simulink model "flatearthsixdof"  (R2025a)
settings: Solver=FixedStepAuto  StartTime=0.0  StopTime=90  FixedStep=0.01  RelTol=1e-3
model workspace (MAT data in the model file):
  aero_data.Mach = [0.01 0.02 0.03 0.04 0.05 0.06 0.07 0.08 0.09 0.1 0.11 0.12 ... (7499 elements, 7499x1)]
  aero_data.Alpha = [0 0 0 0 0 0 0 0 0 0 0 0 ... (7499 elements, 7499x1)]
  aero_data.CD = [0.376420475734 0.37891218399 0.374582423788 0.370163231763 0.366269784455 0.362896739037 0.359959262302 0.357376271103 0.355082207872 0.35302595791 0.351167736032 0.349476360929 ... (7499 elements, 7499x1)]
  aero_data.CL = [0 0 0 0 0 0 0 0 0 0 0 0 ... (7499 elements, 7499x1)]
  aero_data.CP = [3.54714585938 3.54714585938 3.54714585938 3.54714585938 3.54714585938 3.54714585938 3.54714585938 3.54714585938 3.54714585938 3.54714585938 3.54714585938 3.54714585938 ... (7499 elements, 7499x1)]
  aero_data.CNalpha = [4.21136352134 4.21136352134 4.21136352134 4.21136352134 4.21136352134 4.21136352134 4.21136352134 4.21136352134 4.21136352134 4.21136352134 4.21136352134 4.21136352134 ... (7499 elements, 7499x1)]
  aero_data.Cm_alpha = [7.59260560273 7.59260560273 7.59260560273 7.59260560273 7.59260560273 7.59260560273 7.59260560273 7.59260560273 7.59260560273 7.59260560273 7.59260560273 7.59260560273 ... (7499 elements, 7499x1)]
  d_body_mc = 0.4
  designFocus = "reference-tracking"
  drydenSeed_mc = [23341 23342 23343 23344]
  m_initial_mc = [0 20 25 25 20 25 70 1 10 15 1 20 120 1 50 5 1 5 5 10 10]
  schedule(1).Mach_grid = 0
  schedule(1).Kp = 0.0539603522173
  schedule(1).Kd = 0.0467310358173
  schedule(1).Ts = 0.0389337885936
  schedule(2).Mach_grid = 0.1
  schedule(2).Kp = 0.0926620388775
  schedule(2).Kd = 0.0630517482841
  schedule(2).Ts = 0.0389337885936
  schedule(3).Mach_grid = 0.2
  schedule(3).Kp = 0.148668674318
  schedule(3).Kd = 0.0833093726921
  schedule(3).Ts = 0.0389337885936
  schedule(4).Mach_grid = 0.3
  schedule(4).Kp = 0.224059304208
  schedule(4).Kd = 0.106722577169
  schedule(4).Ts = 0.0389337885936
  schedule(5).Mach_grid = 0.4
  schedule(5).Kp = 1.96086663664
  schedule(5).Kd = 0.812163631669
  schedule(5).Ts = 0.0389337885936
  schedule(6).Mach_grid = 0.5
  schedule(6).Kp = 2.40062252085
  schedule(6).Kd = 0.879576960286
  schedule(6).Ts = 0.0389337885936
  schedule(7).Mach_grid = 0.6
  schedule(7).Kp = 2.80522895598
  schedule(7).Kd = 0.92149637698
  schedule(7).Ts = 0.0389337885936
  schedule(8).Mach_grid = 0.7
  schedule(8).Kp = 3.14273502179
  schedule(8).Kd = 0.935580375892
  schedule(8).Ts = 0.0389337885936
  schedule(9).Mach_grid = 0.8
  schedule(9).Kp = 1.01599465816
  schedule(9).Kd = 0.276532829281
  schedule(9).Ts = 0.0389337885936
  schedule(10).Mach_grid = 0.9
  schedule(10).Kp = 3.37328201224
  schedule(10).Kd = 0.845653344317
  schedule(10).Ts = 0.0389337885936
  schedule(11).Mach_grid = 1
  schedule(11).Kp = 2.87563806108
  schedule(11).Kd = 0.668149554703
  schedule(11).Ts = 0.0389337885936
  schedule(12).Mach_grid = 1.1
  schedule(12).Kp = 2.15595228552
  schedule(12).Kd = 0.466777362151
  schedule(12).Ts = 0.0389337885936
  x_mc = [0 0.3 0.7 1.1 1.2 2.2 2.3 2.9 3.1 3.3 3.4 4 4.2 4.3 4.9 6 6.5 6.7 6.9 7.1 7.6]
undefined symbols (not defined in the file or in its folder): F, Light, MIL
libraries: simulink_extras x6, aerolibutil x2, aerolibwind2 x1, aerolibatmos2 x1
settings Model: Creator=rog  LastModifiedBy=rog

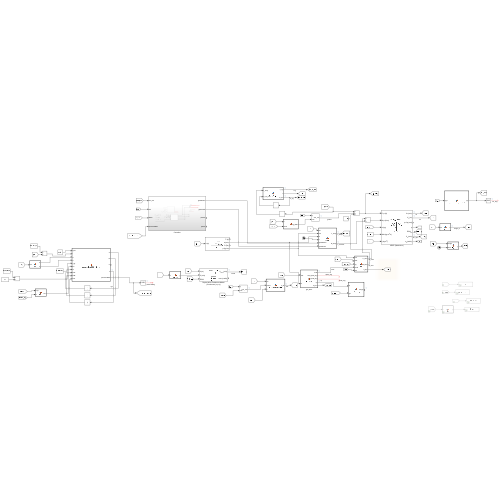
[thumbnail: Simulink's stored preview of the top-level diagram]
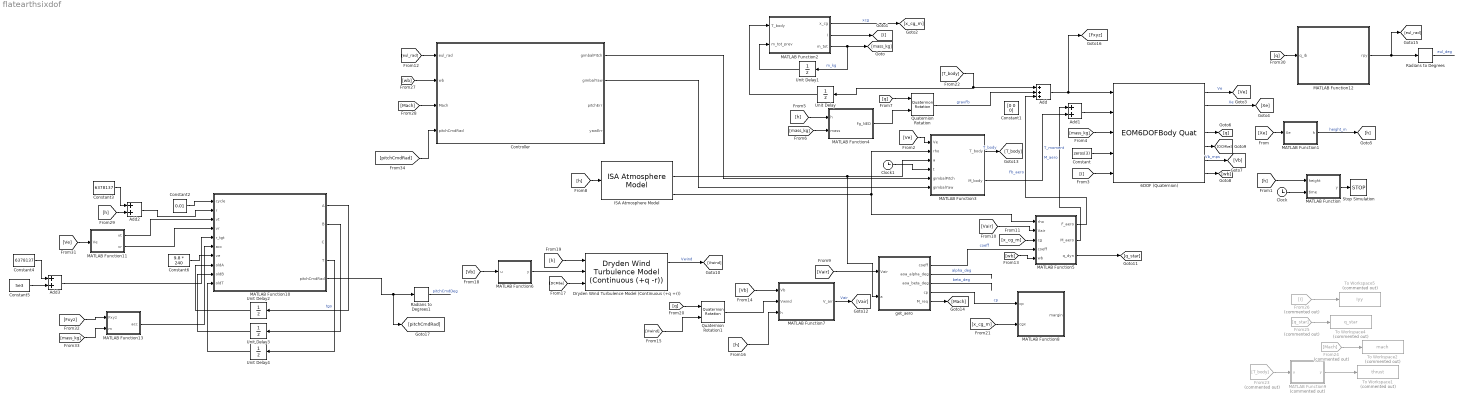
== system flatearthsixdof ==
  6DOF (Quaternion) : EOM6DOFBodyQuat  mtype=Custom Variable  Vm_0=[0.1 0 0]  eul_0=[0 deg2rad(90) 0]
  Add : Sum  Inputs=+++
  Add1 : Sum
  Add2 : Sum
  Add3 : Sum
  Clock : Clock
  Clock1 : Clock
  Constant : Constant  Value=zeros(3)
  Constant1 : Constant  Value=[0 0 0]
  Constant2 : Constant  Value=0.01
  Constant3 : Constant  Value=6378137
  Constant4 : Constant  Value=6378137
  Constant5 : Constant  Value=5e3
  Constant6 : Constant  Value=9.8 * 240
  Controller : Subsystem
  Dryden Wind Turbulence Model (Continuous (+q +r)) : aerolibwind2/Dryden Wind Turbulence Model  (Continuous (+q -r))  units=Metric (MKS)  spec=MIL-F-8785C  model=Continuous Dryden (+q +r)  W20=15  Wdeg=0  TurbProb=10^-2 - Light  L_high=533.4  Wingspan=10  ts=0.1  Seed=drydenSeed_mc  T_on=on
      settings: LibrarySourceBlock=|
      | aerolibwind2/Dryden Wind Turbulence Model
      | (Continuous (+q +r))
  From23 : From  Commented=on  GotoTag=T_body
  From24 : From  Commented=on  GotoTag=Mach
  From25 : From  Commented=on  GotoTag=q_star
  From26 : From  Commented=on  GotoTag=I
  ISA Atmosphere Model : aerolibatmos2/ISA Atmosphere Model  useExtended=on  action=Warning  custom=off  viscosityOut=off  g=9.80665  gamma=1.4  R=287.0531  L=0.0065  h_trop=11000  h_strat=20000  rho0=1.225  P0=101325  T0=288.15  h0=0  S=110.4  Tref=273.15  muref=1.716e-5
  MATLAB Function : MATLAB Function  TreatAsAtomicUnit=on
  MATLAB Function1 : MATLAB Function  TreatAsAtomicUnit=on
  MATLAB Function10 : MATLAB Function  TreatAsAtomicUnit=on
  MATLAB Function11 : MATLAB Function  TreatAsAtomicUnit=on
  MATLAB Function12 : MATLAB Function  TreatAsAtomicUnit=on
  MATLAB Function13 : MATLAB Function  TreatAsAtomicUnit=on
  MATLAB Function2 : MATLAB Function  TreatAsAtomicUnit=on
  MATLAB Function3 : MATLAB Function  TreatAsAtomicUnit=on
  MATLAB Function4 : MATLAB Function  TreatAsAtomicUnit=on
  MATLAB Function5 : MATLAB Function  TreatAsAtomicUnit=on
  MATLAB Function6 : MATLAB Function  TreatAsAtomicUnit=on
  MATLAB Function7 : MATLAB Function  TreatAsAtomicUnit=on
  MATLAB Function8 : MATLAB Function  TreatAsAtomicUnit=on
  MATLAB Function9 : MATLAB Function  Commented=on  TreatAsAtomicUnit=on
  Quaternion Rotation : aerolibutil/Quaternion Rotation
  Quaternion Rotation1 : aerolibutil/Quaternion Rotation
  Radians to Degrees : simulink_extras/Transformations/Radians to Degrees
  Radians to Degrees1 : simulink_extras/Transformations/Radians to Degrees
  Stop Simulation : Stop
  To Workspace1 : ToWorkspace  Commented=on  VariableName=thrust  SaveFormat=Timeseries  SampleTime=-1
  To Workspace2 : ToWorkspace  Commented=on  VariableName=mach  SaveFormat=Timeseries  SampleTime=-1
  To Workspace4 : ToWorkspace  Commented=on  VariableName=q_star  SaveFormat=Timeseries  SampleTime=-1
  To Workspace5 : ToWorkspace  Commented=on  VariableName=Iyy  SaveFormat=Timeseries  SampleTime=-1
  Unit Delay : UnitDelay  InitialCondition=[0 0 0]  SampleTime=-1  HasFrameUpgradeWarning=on
  Unit Delay1 : UnitDelay  InitialCondition=439  SampleTime=-1  HasFrameUpgradeWarning=on
  Unit Delay2 : UnitDelay  SampleTime=-1  HasFrameUpgradeWarning=on
  Unit Delay3 : UnitDelay  SampleTime=-1  HasFrameUpgradeWarning=on
  Unit Delay4 : UnitDelay  InitialCondition=90  SampleTime=-1  HasFrameUpgradeWarning=on
  get_aero : MATLAB Function  TreatAsAtomicUnit=on
  wires:
  Constant/1 -> 6DOF (Quaternion)/4
  MATLAB Function/1(y) -> Stop Simulation/1
  Clock/1 -> MATLAB Function/2(time)
  MATLAB Function2/2(I) -> [I]
  MATLAB Function2/1(x_cg) -> [x_cg_m]  "xcg"
  MATLAB Function2/3(m_tot) -> Unit Delay1/1, [mass_kg]  "m_kg"
  6DOF (Quaternion)/1 -> [Ve]  "Ve"
  6DOF (Quaternion)/2 -> [Xe]  "Xe"
  [h] -> MATLAB Function/1(height)
  [Xe] -> MATLAB Function1/1(Xe)
  MATLAB Function1/1(h) -> [h]  "height_m"
  [Ve] -> MATLAB Function3/1(Ve)
  [I] -> 6DOF (Quaternion)/5
  [mass_kg] -> 6DOF (Quaternion)/3
  Add/1 -> [Fxyz], 6DOF (Quaternion)/1
  [h] -> MATLAB Function4/1(h)
  [mass_kg] -> MATLAB Function4/2(mass)
  6DOF (Quaternion)/4 -> [q]
  [q] -> Quaternion Rotation/1
  MATLAB Function4/1(Fg_NED) -> Quaternion Rotation/2
  Quaternion Rotation/1 -> Add/2  "gravFb"
  [h] -> ISA Atmosphere Model/1
  Clock1/1 -> MATLAB Function3/4(t)
  6DOF (Quaternion)/6 -> [Vb]  "Vb_mps"
  ISA Atmosphere Model/2 -> get_aero/2(a), MATLAB Function3/3(a)
  get_aero/1(coeff) -> MATLAB Function5/4(coeff)  "coeff"
  [x_cg_m] -> MATLAB Function5/3(cg)
  Radians to Degrees/1 -> ?  "eul_deg"
  get_aero/2(aoa_alpha_deg) -> ?  "alpha_deg"
  get_aero/3(aoa_beta_deg) -> ?  "beta_deg"
  [wb] -> MATLAB Function5/5(wb)
  6DOF (Quaternion)/7 -> [wb]
  Unit Delay/1 -> MATLAB Function2/1(T_body)
  ISA Atmosphere Model/4 -> MATLAB Function5/1(rho), MATLAB Function3/2(rho)
  6DOF (Quaternion)/5 -> [DCMbe]
  [h] -> Dryden Wind Turbulence Model (Continuous (+q +r))/1
  MATLAB Function6/1(y) -> Dryden Wind Turbulence Model (Continuous (+q +r))/2
  [DCMbe] -> Dryden Wind Turbulence Model (Continuous (+q +r))/3
  [Vb] -> MATLAB Function6/1(u)
  Dryden Wind Turbulence Model (Continuous (+q +r))/1 -> [Vwind]  "Vwind"
  [Vb] -> MATLAB Function7/1(Vb)
  Quaternion Rotation1/1 -> MATLAB Function7/2(Vwind)
  MATLAB Function7/1(V_air) -> [Vair]  "Vair"
  [Vwind] -> Quaternion Rotation1/2
  [q] -> Quaternion Rotation1/1
  Unit Delay1/1 -> MATLAB Function2/2(m_tot_prev)
  get_aero/4(cp) -> MATLAB Function8/1(cp)  "cp"
  MATLAB Function5/1(F_aero) -> Add/3  "Fb_aero"
  [Vair] -> get_aero/1(Vair)
  [Vair] -> MATLAB Function5/2(Vair)
  [h] -> MATLAB Function7/3(h)
  [x_cg_m] -> MATLAB Function8/2(cgx)
  MATLAB Function5/3(q_dyn) -> [q_star]
  From25/1 -> To Workspace4/1
  From26/1 -> To Workspace5/1
  MATLAB Function3/1(T_body) -> [T_body]  "T_body"
  [T_body] -> Unit Delay/1, Add/1
  From23/1 -> MATLAB Function9/1(u)
  MATLAB Function9/1(y) -> To Workspace1/1
  get_aero/5(M_req) -> [Mach]
  From24/1 -> To Workspace2/1
  Add1/1 -> 6DOF (Quaternion)/2
  MATLAB Function3/2(M_body) -> Add1/2  "T_moment"
  [q] -> MATLAB Function12/1(q_ib)
  MATLAB Function12/1(rpy) -> [eul_rad], Radians to Degrees/1
  MATLAB Function5/2(M_aero) -> Add1/1  "M_aero"
  Controller/1(gimbalPitch) -> MATLAB Function3/5(gimbalPitch)
  Controller/2(gimbalYaw) -> MATLAB Function3/6(gimbalYaw)
  [eul_rad] -> Controller/1(eul_rad)
  [wb] -> Controller/2(wb)
  [Mach] -> Controller/3(Mach)
  MATLAB Function10/1(A) -> Unit Delay2/1
  MATLAB Function10/2(B) -> Unit Delay3/1
  MATLAB Function10/4(T) -> Unit Delay4/1  "tgo"
  Unit Delay4/1 -> MATLAB Function10/10(oldT)
  Unit Delay3/1 -> MATLAB Function10/9(oldB)
  Unit Delay2/1 -> MATLAB Function10/8(oldA)
  Constant2/1 -> MATLAB Function10/1(cycle)
  Constant3/1 -> Add2/1
  [h] -> Add2/2
  Add2/1 -> MATLAB Function10/2(r)
  [Ve] -> MATLAB Function11/1(Ve)
  MATLAB Function11/1(vt) -> MATLAB Function10/3(vt)
  MATLAB Function11/2(vr) -> MATLAB Function10/4(vr)
  Constant5/1 -> Add3/2
  Constant4/1 -> Add3/1
  Add3/1 -> MATLAB Function10/5(r_tgt)
  Constant6/1 -> MATLAB Function10/7(ve)
  [Fxyz] -> MATLAB Function13/1(Fxyz)
  [mass_kg] -> MATLAB Function13/2(m)
  MATLAB Function13/1(acc) -> MATLAB Function10/6(acc)
  MATLAB Function10/5(pitchCmdRad) -> [pitchCmdRad], Radians to Degrees1/1
  Radians to Degrees1/1 -> ?  "pitchCmdDeg"
  [pitchCmdRad] -> Controller/4(pitchCmdRad)

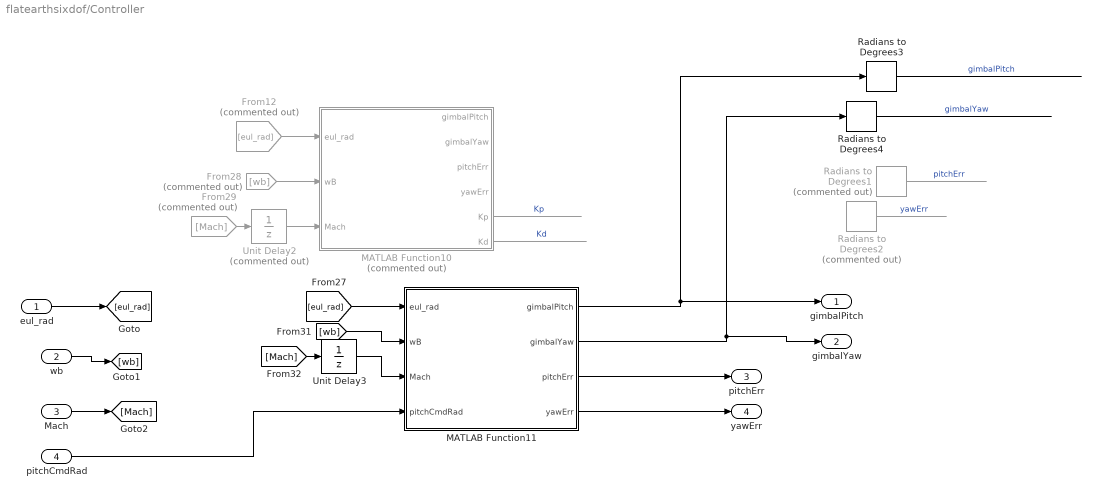
== system flatearthsixdof/Controller ==
  eul_rad : Inport
  wb : Inport  Port=2
  Mach : Inport  Port=3
  pitchCmdRad : Inport  Port=4
  From12 : From  Commented=on  GotoTag=eul_rad
  From28 : From  Commented=on  GotoTag=wb
  From29 : From  Commented=on  GotoTag=Mach
  MATLAB Function10 : MATLAB Function  Commented=on  TreatAsAtomicUnit=on
  MATLAB Function11 : MATLAB Function  TreatAsAtomicUnit=on
  Radians to Degrees1 : simulink_extras/Transformations/Radians to Degrees  Commented=on
  Radians to Degrees2 : simulink_extras/Transformations/Radians to Degrees  Commented=on
  Radians to Degrees3 : simulink_extras/Transformations/Radians to Degrees
  Radians to Degrees4 : simulink_extras/Transformations/Radians to Degrees
  Unit Delay2 : UnitDelay  Commented=on  SampleTime=-1  HasFrameUpgradeWarning=on
  Unit Delay3 : UnitDelay  SampleTime=-1  HasFrameUpgradeWarning=on
  gimbalPitch : Outport
  gimbalYaw : Outport  Port=2
  pitchErr : Outport  Port=3
  yawErr : Outport  Port=4
  wires:
  From28/1 -> MATLAB Function10/2(wB)
  Radians to Degrees1/1 -> ?  "pitchErr"
  From12/1 -> MATLAB Function10/1(eul_rad)
  Radians to Degrees3/1 -> ?  "gimbalPitch"
  [Mach] -> Unit Delay3/1
  Radians to Degrees2/1 -> ?  "yawErr"
  From29/1 -> Unit Delay2/1
  MATLAB Function10/6(Kd) -> ?  "Kd"
  Unit Delay2/1 -> MATLAB Function10/3(Mach)
  [wb] -> MATLAB Function11/2(wB)
  [eul_rad] -> MATLAB Function11/1(eul_rad)
  MATLAB Function11/2(gimbalYaw) -> Radians to Degrees4/1, gimbalYaw/1
  Unit Delay3/1 -> MATLAB Function11/3(Mach)
  Radians to Degrees4/1 -> ?  "gimbalYaw"
  MATLAB Function11/4(yawErr) -> yawErr/1
  MATLAB Function10/5(Kp) -> ?  "Kp"
  MATLAB Function11/3(pitchErr) -> pitchErr/1
  Mach/1 -> [Mach]
  wb/1 -> [wb]
  eul_rad/1 -> [eul_rad]
  pitchCmdRad/1 -> MATLAB Function11/4(pitchCmdRad)
  MATLAB Function11/1(gimbalPitch) -> gimbalPitch/1, Radians to Degrees3/1

== matlab function flatearthsixdof/MATLAB Function6 ==
  data: u input; y output
function y = twonorm(u)

y = norm(u);

== matlab function flatearthsixdof/get_aero ==
  data: Vair input size=[3 1]; coeff output; a input; aoa_alpha_deg output; aoa_beta_deg output; cp output; M_req output
function [coeff, aoa_alpha_deg, aoa_beta_deg, cp, M_req] = get_aero(Vair, a)

    u = Vair(1);
    v = Vair(2);
    w = Vair(3);

    V = sqrt(u*u + v*v + w*w);

    if V < 1e-6
        coeff = zeros(4,1);
        aoa_alpha_deg = 0;
        aoa_beta_deg  = 0;
        cp = 0;
        M_req = 0;
        return;
    end

    % Alpha / beta
    alpha = atan2(w, u);
    Vxz   = sqrt(u*u + w*w);

    if Vxz < 1e-6
        beta = 0;
    else
        beta = atan2(v, Vxz);
    end

    alpha_deg = alpha * 180/pi;
    beta_deg  = beta  * 180/pi;

    aoa_alpha_deg = alpha_deg;
    aoa_beta_deg  = beta_deg;

    % Total angle for drag & CP
    alpha_t = atan2( sqrt(v*v + w*w), u );
    aoa_t_deg = alpha_t * 180/pi;

    M_req = V / a;

    % Load aero once
    persistent aero
    if isempty(aero)
        S = load("aero.mat");
        aero = S.aero_data;
    end

    Alpha   = aero.Alpha;
    Mach    = aero.Mach;
    CD_full = aero.CD;
    CL_full = aero.CL;
    CP_full = aero.CP;

    % Lift from alpha & beta (same symmetric table)
    [~, CLa, ~] = lookup_coeff_nearest(alpha_deg, M_req, Alpha, Mach, CD_full, CL_full, CP_full);
    [~, CLb, ~] = lookup_coeff_nearest(beta_deg,  M_req, Alpha, Mach, CD_full, CL_full, CP_full);

    % Drag + CP from total angle
    [CD, ~, CP] = lookup_coeff_nearest(aoa_t_deg, M_req, Alpha, Mach, CD_full, CL_full, CP_full);

    cp = CP;

    coeff = [CD; CLa; CLb; CP];
end


function [cd, cl, cp] = lookup_coeff(aoa_deg, M_req, ...
                                     Alpha, Mach, CD_full, CL_full, CP_full)

    [~, iMach] = min(abs(Mach - M_req));
    Mach_near  = Mach(iMach);

    rows = find(abs(Mach - Mach_near) < 1e-6);

    A_slice  = Alpha(rows);
    CD_slice = CD_full(rows);
    CL_slice = CL_full(rows);
    CP_slice = CP_full(rows);

    cd = interp1(A_slice, CD_slice, aoa_deg, "linear", "extrap");
    cl = interp1(A_slice, CL_slice, aoa_deg, "linear", "extrap");
    cp = interp1(A_slice, CP_slice, aoa_deg, "linear", "extrap");
end


function [cd, cl, cp] = lookup_coeff_nearest(aoa_deg, M_req, ...
                                             Alpha, Mach, CD_full, CL_full, CP_full)

    [~, iMach] = min(abs(Mach - M_req));
    Mach_near  = Mach(iMach);

    rows = find(abs(Mach - Mach_near) < 1e-6);

    A_slice = Alpha(rows);

    [~, k] = min(abs(A_slice - aoa_deg));
    idx    = rows(k);

    cd = CD_full(idx);
    cl = CL_full(idx);
    cp = CP_full(idx);
end

== matlab function flatearthsixdof/MATLAB Function8 ==
  data: cp input; margin output; cgx input; d_body_mc parameter
function margin  = stabilitymargin(cp, cgx, d_body_mc)


margin = (cp-cgx)/d_body_mc;

== matlab function flatearthsixdof/MATLAB Function9 ==
  data: u input; y output
function y = fcn(u)

y = norm(u);

== matlab function flatearthsixdof/Controller/MATLAB Function10 ==
  data: eul_rad input; gimbalPitch output; wB input; Mach input; gimbalYaw output; pitchErr output; yawErr output; schedule parameter; Kp output; Kd output
function [gimbalPitch, gimbalYaw, pitchErr, yawErr, Kp, Kd] = tvc_gainsched_eulXYZ_pd(eul_rad, wB, Mach, schedule)
% Gain-scheduled TVC PD controller using Euler attitude error (XYZ order).
% eul_rad is assumed to be Euler angles RELATIVE TO THE VERTICAL reference,
% so the desired attitude corresponds to eul_rad = [0;0;0] (or [0 0 0]).
%
% Euler order: XYZ
%   eul_rad(1) = roll  about body +X
%   eul_rad(2) = pitch about body +Y
%   eul_rad(3) = yaw   about body +Z
%
% Control uses pitch and yaw only:
%   pitchErr = eul_rad(2), yawErr = eul_rad(3)
% D term uses measured body rates:
%   q_rate = wB(2), r_rate = wB(3)

%% ----- USER LIMITS -----
gimbalLimit = deg2rad(6);

%% ----- Gain schedule (nearest Mach) -----
n = numel(schedule);
Mach_grid = zeros(n,1);
Kp_table  = zeros(n,1);
Kd_table  = zeros(n,1);

for i = 1:n
    Mach_grid(i) = schedule(i).Mach_grid;
    Kp_table(i)  = schedule(i).Kp;
    Kd_table(i)  = schedule(i).Kd;
end

idx = nearestIndex(Mach_grid, Mach);
Kp = Kp_table(idx);
Kd = Kd_table(idx);

%% ----- Attitude errors from Euler error angles -----
% Ensure column vector indexing works either way
eul_rad = eul_rad(:);

% XYZ: [roll; pitch; yaw]
pitchErr = eul_rad(2);   % about body-Y
yawErr   = eul_rad(3);   % about body-Z

%% ----- Body rates for D term -----
q_rate = wB(2);          % pitch rate about body-Y
r_rate = wB(3);          % yaw rate about body-Z

%% ----- PD control law -----
% Sign chosen so positive error / positive rate yields gimbal that creates restoring moment
gimbalPitch = (Kp*pitchErr + Kd*q_rate);
gimbalYaw   = (Kp*yawErr   + Kd*r_rate);

%% ----- Saturation -----
gimbalPitch = min(max(gimbalPitch, -gimbalLimit), gimbalLimit);
gimbalYaw   = min(max(gimbalYaw,   -gimbalLimit), gimbalLimit);

end

%% ===== Helper: nearest index =====
function idx = nearestIndex(x, xq)
    [~, idx] = min(abs(x - xq));
end

== matlab function flatearthsixdof/Controller/MATLAB Function11 ==
  data: eul_rad input; gimbalPitch output; wB input; Mach input; gimbalYaw output; pitchErr output; yawErr output; schedule parameter; pitchCmdRad input
function [gimbalPitch, gimbalYaw, pitchErr, yawErr] = tvc_gainsched_eulXYZ_lqr(eul_rad, wB, Mach, schedule, pitchCmdRad)
% Gain-scheduled TVC "LQR-style" controller using Euler error angles (XYZ).
% eul_rad is relative-to-vertical error, so desired = [0;0;0].
%pitchCmdRad = 0;
gimbalLimit = deg2rad(6);

% ----- Nearest Mach lookup -----
n = numel(schedule);
Mach_grid = zeros(n,1);
K_table   = zeros(n,2);

for i = 1:n
    Mach_grid(i) = schedule(i).Mach_grid;
    K_table(i,:) = schedule(i).Kd;   % [K_theta  K_rate]
end

idx = nearestIndex(Mach_grid, Mach);
K = K_table(idx,:);

% ----- Errors -----
eul_rad = eul_rad(:);      % force column
pitchErr = eul_rad(2) - pitchCmdRad;     % about body-Y
yawErr   = eul_rad(3);     % about body-Z

% ----- Rates -----
q_rate = wB(2);
r_rate = wB(3);

% ----- Control (sign matches restoring moments) -----
gimbalPitch = (K(1)*pitchErr + K(2)*q_rate);
gimbalYaw   = (K(1)*yawErr   + K(2)*r_rate);

% ----- Saturation -----
gimbalPitch = min(max(gimbalPitch, -gimbalLimit), gimbalLimit);
gimbalYaw   = min(max(gimbalYaw,   -gimbalLimit), gimbalLimit);

end

function idx = nearestIndex(x, xq)
    [~, idx] = min(abs(x - xq));
end

== matlab function flatearthsixdof/MATLAB Function12 ==
  data: q_ib input; rpy output
function rpy = qib_to_rpy_vs_vertical(q_ib)
% q_ib_to_rpy_vs_vertical
% q_ib: quaternion (i -> b), NED inertial, scalar-first [w x y z]'
% rpy: [roll; pitch; yaw] in radians, relative to "vertical/up"

% ---- Normalize quaternion ----
q = q_ib(:);
q = q ./ max(1e-12, norm(q));

q0 = q(1); q1 = q(2); q2 = q(3); q3 = q(4);

% ---- Quaternion to DCM (i -> b) ----
C_ib = [ ...
    1-2*(q2^2+q3^2),   2*(q1*q2+q0*q3),   2*(q1*q3-q0*q2); ...
    2*(q1*q2-q0*q3),   1-2*(q1^2+q3^2),   2*(q2*q3+q0*q1); ...
    2*(q1*q3+q0*q2),   2*(q2*q3-q0*q1),   1-2*(q1^2+q2^2)  ];

% ---- Define "vertical frame" v in inertial NED ----
% x_v = Up, y_v = East, z_v = North (right-handed)
xv_i = [0; 0; -1];
yv_i = [0; 1;  0];
zv_i = [1; 0;  0];

% DCM (i -> v): rows are v-axes expressed in i
C_iv = [xv_i.'; yv_i.'; zv_i.'];

% We want C_vb = (v -> b) = (i -> b) * (v -> i)
C_vi = C_iv.';          % (v -> i)
C_vb = C_ib * C_vi;     % (v -> b)

% ---- DCM to Euler 3-2-1 (roll-pitch-yaw) ----
% Using same 3-2-1 convention as standard aerospace DCM:
% C(1,3) = -sin(theta)
c13 = C_vb(1,3);
c13 = min(1, max(-1, c13));   % numeric safety

pitch = asin(-c13);
roll  = atan2(C_vb(2,3), C_vb(3,3));
yaw   = atan2(C_vb(1,2), C_vb(1,1));

rpy = [roll; pitch; yaw];
end

== matlab function flatearthsixdof/MATLAB Function10 ==
  data: cycle input; A output; r input; vt input; vr input; r_tgt input; acc input; ve input; oldA input; oldB input; oldT input; B output; C output; T output; pitchCmdRad output
function [A,B,C,T,pitchCmdRad] = poweredExplicitGuidance(cycle, r, vt, vr, r_tgt, acc, ve, oldA, oldB, oldT)
%#codegen
% r and r_tgt are RADII from body center [m]

mu = 3.986004418e14;  % [m^3/s^2] Earth

% guards
acc = max(acc, 1e-3);
oldT = max(oldT, 1e-3);

tau = ve / acc;

% If oldA/oldB uninitialized, estimate from oldT
if oldA==0 && oldB==0
    Tuse = min(oldT, 0.999*tau);
    b0 = -ve*log(1 - Tuse/tau);
    b1 = b0*tau - ve*Tuse;
    c0 = b0*Tuse - b1;
    c1 = c0*tau - ve*Tuse^2/2;

    matA = [b0 b1; c0 c1];
    matB = [-vr; r_tgt - r - vr*Tuse];
    x = matA \ matB;
    oldA = x(1); oldB = x(2);
end

% Angular momentum (planar)
angM = r * vt;
tgtV = sqrt(mu / r_tgt);
tgtM = r_tgt * tgtV;
dMom = tgtM - angM;

% Steering series
C_tgt = (mu/r_tgt^2 - tgtV^2/r_tgt) / (acc/(1 - min(oldT,0.999*tau)/tau));
f_r_T = oldA + oldB*oldT + C_tgt;

C = (mu/r^2 - vt^2/r) / acc;
f_r = oldA + C;
f_r_dot = (f_r_T - f_r) / oldT;

f_theta = 1 - f_r^2/2;
f_theta_dot = -f_r*f_r_dot;
f_theta_2dot = -f_r_dot^2/2;

avgR = 0.5*(r + r_tgt);
deltav = dMom/avgR + ve*(oldT-cycle)*(f_theta_dot+f_theta_2dot*tau) + f_theta_2dot*ve*(oldT-cycle)^2/2;
deltav = deltav / (f_theta + f_theta_dot*tau + f_theta_2dot*tau^2);

T = tau*(1 - exp(-deltav/ve));
T = max(T, 0.0);
T = min(T, 0.999*tau);

if T >= 7.5
    b0 = -ve*log(1 - T/tau);
    b1 = b0*tau - ve*T;
    c0 = b0*T - b1;
    c1 = c0*tau - ve*T^2/2;

    matA = [b0 b1; c0 c1];
    matB = [-vr; r_tgt - r - vr*T];
    x = matA \ matB;

    A = x(1); B = x(2);
else
    A = oldA; B = oldB;
end

A = min(max(A,-1.0),1.0);
pitchCmdRad = acos(A);

end

== matlab function flatearthsixdof/MATLAB Function11 ==
  data: Ve input; vt output; vr output
function [vt, vr]  = fcn(Ve)

vt = Ve(1);
vr = -Ve(3);

== matlab function flatearthsixdof/MATLAB Function13 ==
  data: Fxyz input; acc output; m input
function acc = fcn(Fxyz, m)

acc = norm(Fxyz)/m;

== matlab function flatearthsixdof/MATLAB Function2 ==
  data: x_cg output; I output; m_tot output; T_body input; m_tot_prev input; x_mc parameter; m_initial_mc parameter
function [x_cg, I, m_tot] = MassProps(T_body, m_tot_prev, x_mc, m_initial_mc)

    x = x_mc;
    m_initial = m_initial_mc;
    d = 0.4;

    persistent m0 x_cg0 Ixx0 Iyy0 initialized
    if isempty(initialized)
        m0    = sum(m_initial);
        x_cg0 = sum(m_initial .* x) / m0;

        r    = x - x_cg0;
        Iyy0 = sum(m_initial .* r.^2);
        Ixx0 = 0.5 * m0 * (d/2)^2;

        initialized = true;
    end

    g0  = 9.80665;
    Isp = 240;
    Ts  = 0.01;

    Tmag = abs(T_body(1));
    if Isp > 0
        mdot = Tmag / (Isp * g0);
    else
        mdot = 0;
    end

    m_tot = m_tot_prev - mdot * Ts;
    if m_tot < 0
        m_tot = 0;
    end

    x_cg = 7.6 - x_cg0;

    if m0 > 0
        scale = m_tot / m0;
    else
        scale = 0;
    end

    Ixx = Ixx0 * scale;
    Iyy = Iyy0 * scale;

    I = [Ixx 0   0;
         0   Iyy 0;
         0   0   Iyy];
end

== matlab function flatearthsixdof/MATLAB Function1 ==
  data: Xe input; h output
function h = fcn(Xe)

h = -Xe(3);

== matlab function flatearthsixdof/MATLAB Function ==
  data: height input; time input; y output
function y = fcn(height, time)

if time > 10 && height < 0
    y = 1;
else
    y = 0;
end

== matlab function flatearthsixdof/MATLAB Function4 ==
  data: h input; Fg_NED output; mass input
function Fg_NED = grav(h, mass)

R = 6378137;

g = 9.80665 * (R/(R + h))^2;

Fg_NED = [0; 0; mass*g];
end

== matlab function flatearthsixdof/MATLAB Function3 ==
  data: Ve input; T_body output size=[1 3]; rho input; a input; t input; gimbalPitch input; gimbalYaw input; M_body output
function [T_body, M_body] = thrust(Ve, rho, a, t, gimbalPitch, gimbalYaw)

    %% ----- USER CONSTANT -----
    ell = 3.3317;   % [m] engine distance behind CG (positive)
    %% -------------------------

    V = norm(Ve);

    % ----- Thrust magnitude model (unchanged) -----
    T_SL = 15.5e3;
    rho0 = 1.225;
    n    = 0.7;
    k_M  = 0.3;

    if a > 0
        M = V / a;
    else
        M = 0;
    end

    sigma = rho / rho0;
    T = T_SL * sigma^n * (1 - k_M * M);

    if T < 0
        T = 0;
    end

    if t > 90 || T == 0
        T_body = [0 0 0];
        M_body = [0 0 0];
        return;
    end

    %% ----- TVC: thrust direction in BODY frame -----
    % Nominal thrust direction (+X body)
    ex = [1; 0; 0];

    cp = cos(gimbalPitch);  sp = sin(gimbalPitch);
    cy = cos(gimbalYaw);    sy = sin(gimbalYaw);

    % Pitch rotation about +Y
    Ry = [ cp  0  sp;
            0  1   0;
          -sp  0  cp];

    % Yaw rotation about +Z
    Rz = [ cy -sy  0;
           sy  cy  0;
            0   0  1];

    % Apply pitch then yaw
    dir_b = Rz * Ry * ex;

    %% ----- Thrust force -----
    F_b = T * dir_b;     % [N], column vector
    T_body = F_b.';      % return as row (Simulink friendly)

    %% ----- Thrust moment about CG -----
    % Engine location vector from CG (aft along -X)
    r_b = [-ell; 0; 0];

    % Moment = r x F
    M_b = cross(r_b, F_b);
    M_body = M_b.';      % row vector

end

== matlab function flatearthsixdof/MATLAB Function5 ==
  data: rho input; Vair input size=[3 1]; cg input; F_aero output; coeff input; M_aero output size=[1 3]; wb input; d_body_mc parameter; q_dyn output
function [F_aero, M_aero, q_dyn] = fcn(rho, Vair, cg, coeff, wb, d_body_mc)



    CD = coeff(1);
    CLa = coeff(2);
    CLb = coeff(3);
    CP  = coeff(4);

    u = Vair(1);
    v = Vair(2);
    w = Vair(3);

    V = sqrt(u*u + v*v + w*w);

    p = wb(1);
    q = wb(2);
    r = wb(3);
 
    % Angles
    alpha = atan2(w, u);
    Vxz   = sqrt(u*u + w*w);

    if Vxz < 1e-6
        beta = 0;
    else
        beta = atan2(v, Vxz);
    end

    Sref  = pi * (d_body_mc/2)^2;
    q_dyn = 0.5 * rho * V * V;

    % Wind-axis forces
    D  = q_dyn * CD  * Sref;
    Lz = q_dyn * CLa * Sref;
    Ly = q_dyn * CLb * Sref;

    Fx_w = -D;
    Fy_w =  Ly;
    Fz_w = -Lz;

    % Wind -> body rotation (Aerospace Blockset convention)
    cA = cos(alpha); sA = sin(alpha);
    cB = cos(beta);  sB = sin(beta);

    Cb_w = [ cA*cB,  -cA*sB, -sA;
              sB,     cB,     0;
             sA*cB,  -sA*sB,  cA ];

    Fb = Cb_w * [Fx_w; Fy_w; Fz_w];

    Fx_b = Fb(1);
    Fy_b = Fb(2);
    Fz_b = Fb(3);

    % Moment from single CP
    rx = CP - cg;

    Mx_b = 0;
    My_b = -rx * Fz_b;
    Mz_b =  rx * Fy_b;

    F_aero = [Fx_b Fy_b Fz_b];
    M_aero = [Mx_b My_b Mz_b];
end

== matlab function flatearthsixdof/MATLAB Function7 ==
  data: Vb input; V_air output; Vwind input; h input
function V_air = effectiveAirspeed(Vb, Vwind, h)

    if h > 10
        V_air = Vb - Vwind;
    else
        V_air = Vb;
    end
    %V_air = Vb;
end
